simulink model "MobileManipulatorSlave"  (R2016a)
settings: Solver=FixedStepAuto  SolverMode=SingleTasking  StartTime=0.0  StopTime=inf  FixedStep=.001  RelTol=1e-3
undefined symbols (not defined in the file): DiscIntNeverNeededParam, transl
libraries: simulink x20, LibrarySimulinkSAS x2, dspfactors x1, aerolibanimutils x1, dspnetwork x1
(part 1 of 2)
settings Model: xpc_rtwmakecfg_data=_jpeg_  Creator=DSANTIAGO  LastModifiedBy=santd
settings DataIOCC: LimitDataPoints=on  SaveFormat=Array
settings OptimizationCC: BlockReduction=off  BooleanDataType=off
settings DebuggingCC: SaveWithParameterizedLinksMsg=none  UnderspecifiedInitializationDetection=Classic  MergeDetectMultiDrivingBlocksExec=none  SignalResolutionControl=TryResolveAllWithWarning  InvalidFcnCallConnMsg=warning  FcnCallInpInsideContextMsg=EnableAllAsWarning
settings HardwareCC: ProdBitPerPointer=32  ProdLargestAtomicFloat=None  ProdIntDivRoundTo=Undefined  ProdEndianess=Unspecified  ProdWordSize=32  ProdHWDeviceType=32-bit Generic  TargetUnknown=on
settings ModelReferenceCC: PropagateSignalLabelsOutOfModel=off
settings ConfigComp: CovSFcnEnable=off

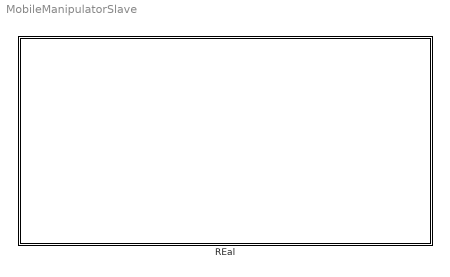
== system MobileManipulatorSlave ==
  "REal " : Subsystem  mask{sel=1, offSet=[1.5e-1 0 0.1]', h1=.01, h2=.01, kgmb=diag([8 10]), kgms=diag([4 4 4]), kms=10, kmb=5, ksb=1, ksm=diag([1 1 1])*2e3}
      mask prompts: sel "Control (s/m)"; h1 "Delay1"; h2 "Delay2"

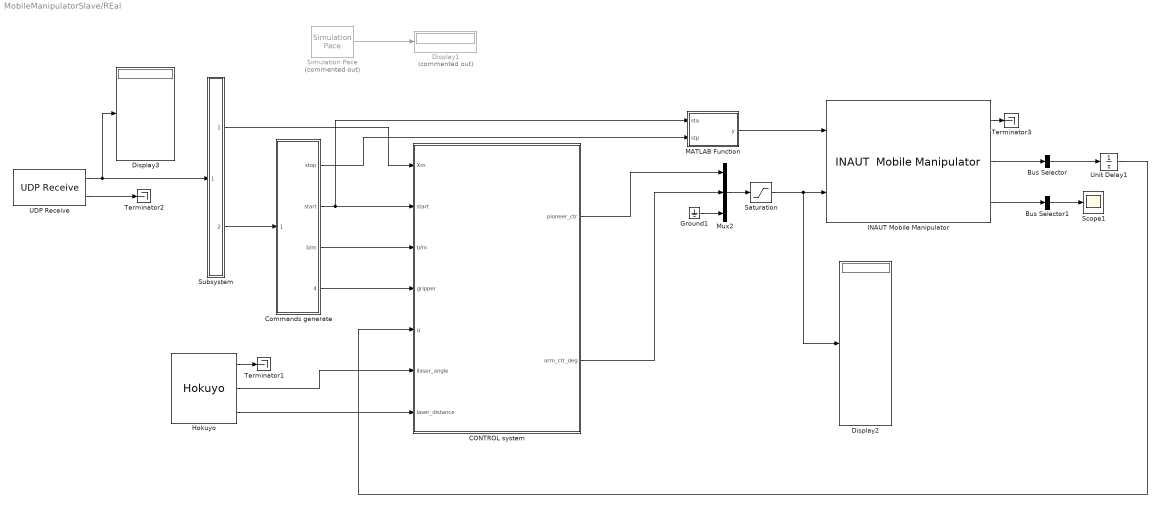
== system MobileManipulatorSlave/REal  ==
  Bus Selector : BusSelector  OutputSignals=q_{arm}  OutputAsBus=on
  Bus Selector1 : BusSelector  OutputSignals=base Info.current rigth motor?,base Info.current left motor?  OutputAsBus=on
  CONTROL system : Subsystem
  Commands generate : Subsystem
  Display1 : Display  Commented=on
  Display2 : Display
  Display3 : Display
  Ground1 : Ground
  Hokuyo : LibrarySimulinkSAS/Hokuyo
  INAUT Mobile Manipulator : LibrarySimulinkSAS/INAUT  Mobile Manipulator  IdB=3  IdM=1  IdL=0  ts=-1
  MATLAB Function : MATLAB Function  TreatAsAtomicUnit=on
  Mux2 : Mux  Inputs=3
  Saturation : Saturate  UpperLimit=2000  LowerLimit=-2000
  Scope1 : Scope
  Simulation Pace : aerolibanimutils/Simulation Pace  Commented=on  SimulationPace=1  SleepMode=MATLAB Thread  OutputPaceError=on  SampleTime=-1
  Subsystem : Subsystem
  Terminator1 : Terminator
  Terminator2 : Terminator
  Terminator3 : Terminator
  UDP Receive : dspnetwork/UDP Receive  localURL='0.0.0.0'  localPort=24100  remoteURL='0.0.0.0'  remotePort=-1  recvBufferSize=1024  dims=7  signalDatatype=double  isVarSize=off  showBlockingTime=off  blockingTime=0  sampletime=-1  blockPlatform=[]
  Unit Delay1 : UnitDelay  SampleTime=-1
  wires:
  Subsystem/1(xm) -> CONTROL system/1(Xm)
  Unit Delay1/1 -> CONTROL system/5(q)
  Subsystem/2(bt) -> Commands generate/1(butons)
  Commands generate/2(start) -> CONTROL system/2(start), MATLAB Function/1(sta)
  CONTROL system/2(arm_ctr_deg) -> Mux2/2
  Mux2/1 -> Saturation/1
  INAUT Mobile Manipulator/2 -> Bus Selector/1
  INAUT Mobile Manipulator/3 -> Bus Selector1/1
  INAUT Mobile Manipulator/1 -> Terminator3/1
  Bus Selector/1 -> Unit Delay1/1
  CONTROL system/1(pioneer_ctr) -> Mux2/1
  Ground1/1 -> Mux2/3
  Simulation Pace/1 -> Display1/1
  Commands generate/3(b/m) -> CONTROL system/3(b/m)
  Commands generate/4(griper) -> CONTROL system/4(gripper)
  UDP Receive/1 -> Subsystem/1(u), Display3/1
  UDP Receive/2 -> Terminator2/1
  Saturation/1 -> Display2/1, INAUT Mobile Manipulator/2
  Bus Selector1/1 -> Scope1/1
  MATLAB Function/1(y) -> INAUT Mobile Manipulator/1
  Commands generate/1(stop) -> MATLAB Function/2(stp)
  Hokuyo/1 -> Terminator1/1
  Hokuyo/2 -> CONTROL system/6(llaser_angle)
  Hokuyo/3 -> CONTROL system/7(laser_distance)

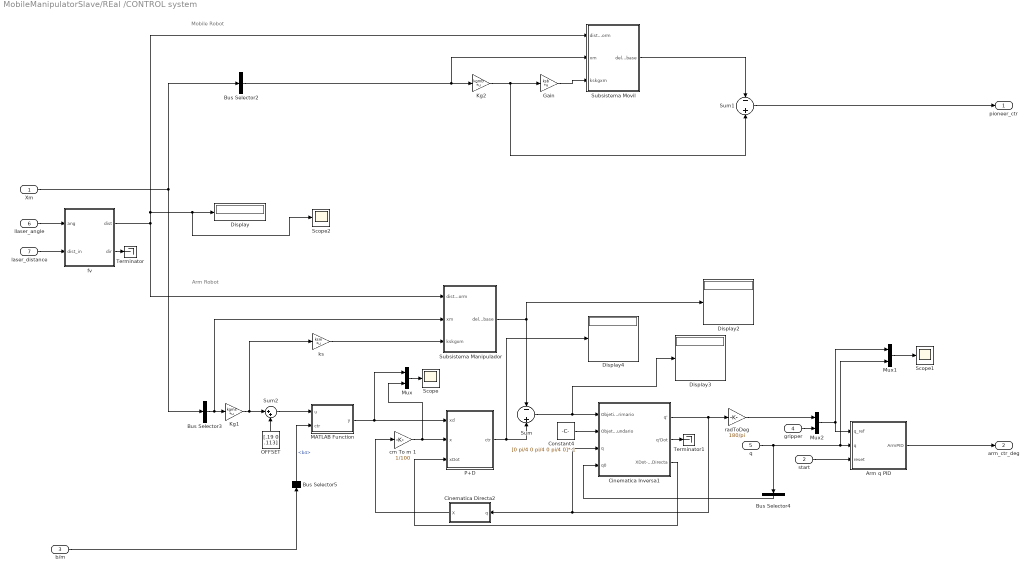
== system MobileManipulatorSlave/REal /CONTROL system ==
  note: Mobile Robot
  note: Arm Robot
  Xm : Inport
  start : Inport  Port=2
  b/m : Inport  Port=3
  gripper : Inport  Port=4
  q : Inport  Port=5
  llaser_angle : Inport  Port=6
  laser_distance : Inport  Port=7
  Arm q PID : Subsystem
  Bus Selector2 : BusSelector  OutputSignals=x,y  OutputAsBus=on
  Bus Selector3 : BusSelector  OutputSignals=x,y,z  OutputAsBus=on
  Bus Selector4 : BusSelector  OutputSignals=q1,q2,q3,q4,q5,q6,q7  OutputAsBus=on
  Bus Selector5 : BusSelector  OutputSignals=b4
  Cinematica Directa2 : Subsystem
  Cinematica Inversa1 : Subsystem
  Constant4 : Constant  Value=[0 pi/4 0 pi/4 0 pi/4 0]*-1
  Display{,2..4} (4 alike) : Display
  Gain : Gain  Gain=ksb  Multiplication=Matrix(K*u)
  Kg1 : Gain  Gain=kgms  Multiplication=Matrix(K*u)
  Kg2 : Gain  Gain=kgmb  Multiplication=Matrix(K*u)
  MATLAB Function : MATLAB Function  TreatAsAtomicUnit=on
  Mux : Mux  Inputs=2
  Mux1 : Mux  Inputs=2
  Mux2 : Mux  Inputs=2
  OFFSET : Constant  Value=[.19 0 .113]
  P+D : Subsystem
  Scope : Scope
  Scope1 : Scope
  Scope2 : Scope
  Subsistema Manipulador : Subsystem
  Subsistema Movil : Subsystem
  Sum : Sum  Inputs=-+
  Sum1 : Sum  Inputs=-+
  Sum2 : Sum  Inputs=|++
  Terminator : Terminator
  Terminator1 : Terminator
  cm To m 1 : Gain  Gain=1/100
  fv : Subsystem
  ks : Gain  Gain=ksm  Multiplication=Matrix(K*u)
  radToDeg : Gain  Gain=180/pi
  pioneer_ctr : Outport
  arm_ctr_deg : Outport  Port=2
  wires:
  Xm/1 -> Bus Selector3/1, Bus Selector2/1
  Bus Selector2/1 -> Subsistema Movil/2(xm), Kg2/1
  Cinematica Inversa1/1(q') -> Cinematica Inversa1/3(q), Cinematica Directa2/1(q), radToDeg/1
  OFFSET/1 -> Sum2/2
  Kg1/1 -> ks/1, Sum2/1
  P+D/1(ctr) -> Display4/1, Sum/2
  Cinematica Directa2/1("X ") -> cm To m 1/1
  cm To m 1/1 -> Mux/2, P+D/2(x)
  Constant4/1 -> Cinematica Inversa1/2(Objetivo Secundario)
  gripper/1 -> Mux2/2
  start/1 -> Arm q PID/3(reset)
  b/m/1 -> Bus Selector5/1
  Kg2/1 -> Sum1/2, Gain/1
  radToDeg/1 -> Mux2/1
  Sum2/1 -> MATLAB Function/1(u)
  Cinematica Inversa1/2(q'Dot) -> Terminator1/1
  Mux/1 -> Scope/1
  Cinematica Inversa1/3(XDot- CinematicaDirecta) -> P+D/3(xDot)
  q/1 -> Bus Selector4/1, Mux1/2, Arm q PID/2(q)
  Mux2/1 -> Mux1/1, Arm q PID/1(q_ref)
  Mux1/1 -> Scope1/1
  Bus Selector4/1 -> Cinematica Inversa1/4(q0)
  MATLAB Function/1(y) -> P+D/1(xd), Mux/1
  Bus Selector5/1 -> MATLAB Function/2(ctr)  "<b4>"
  Arm q PID/1(ArmPID) -> arm_ctr_deg/1
  Gain/1 -> Subsistema Movil/3(kskgxm)
  Subsistema Movil/1(delta_base) -> Sum1/1
  fv/2(dir) -> Terminator/1
  laser_distance/1 -> fv/2(dist_in)
  llaser_angle/1 -> fv/1(ang)
  fv/1(dist) -> Subsistema Manipulador/1(dist_norm), Scope2/1, Display/1, Subsistema Movil/1(dist_norm)
  Subsistema Manipulador/1(delta_base) -> Display2/1, Sum/1
  Sum/1 -> Display3/1, Cinematica Inversa1/1(Objetivo Primario)
  Bus Selector3/1 -> Subsistema Manipulador/2(xm), Kg1/1
  ks/1 -> Subsistema Manipulador/3(kskgxm)
  Sum1/1 -> pioneer_ctr/1

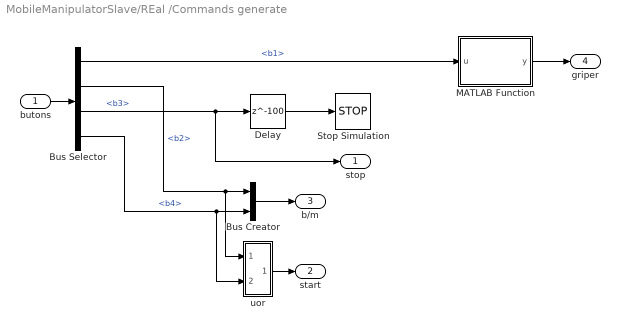
== system MobileManipulatorSlave/REal /Commands generate ==
  butons : Inport
  Bus Creator : BusCreator  Inputs=2
  Bus Selector : BusSelector  OutputSignals=b1,b2,b3,b4
  Delay : Delay  DelayLength=100
  MATLAB Function : MATLAB Function  TreatAsAtomicUnit=on
  Stop Simulation : Stop
  uor : Subsystem
  stop : Outport
  start : Outport  Port=2
  b/m : Outport  Port=3
  griper : Outport  Port=4
  wires:
  Bus Selector/2 -> uor/1(u1), Bus Creator/1  "<b2>"
  Bus Selector/3 -> stop/1, Delay/1  "<b3>"
  Delay/1 -> Stop Simulation/1
  Bus Creator/1 -> b/m/1
  Bus Selector/4 -> uor/2(u2), Bus Creator/2  "<b4>"
  Bus Selector/1 -> MATLAB Function/1(u)  "<b1>"
  butons/1 -> Bus Selector/1
  uor/1(y) -> start/1
  MATLAB Function/1(y) -> griper/1

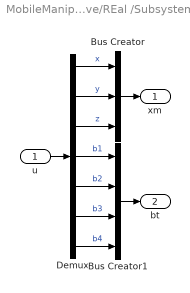
== system MobileManipulatorSlave/REal /Subsystem ==
  u : Inport
  Bus Creator : BusCreator  Inputs=3
  Bus Creator1 : BusCreator  Inputs=4
  Demux : Demux  Outputs=7
  xm : Outport
  bt : Outport  Port=2
  wires:
  Demux/2 -> Bus Creator/2  "y"
  Demux/3 -> Bus Creator/3  "z"
  Demux/5 -> Bus Creator1/2  "b2"
  Demux/1 -> Bus Creator/1  "x"
  Demux/6 -> Bus Creator1/3  "b3"
  Demux/4 -> Bus Creator1/1  "b1"
  Demux/7 -> Bus Creator1/4  "b4"
  Bus Creator1/1 -> bt/1
  u/1 -> Demux/1
  Bus Creator/1 -> xm/1

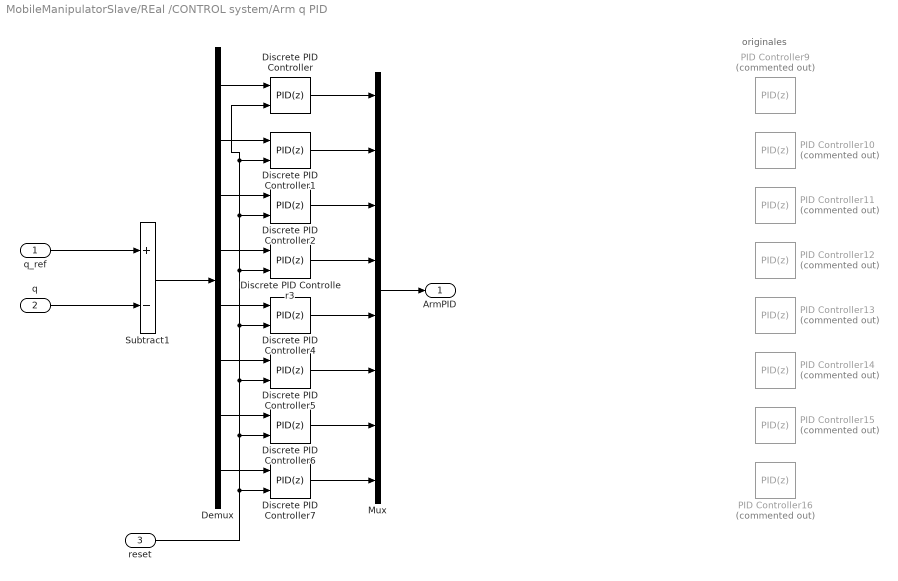
== system MobileManipulatorSlave/REal /CONTROL system/Arm q PID ==
  note: originales
  q_ref : Inport
  q : Inport  Port=2
  reset : Inport  Port=3
  Demux : Demux  Outputs=8
  Discrete PID Controlle r3 : simulink/Continuous/PID Controller  Controller=PID  TimeDomain=Discrete-time  SampleTime=-1  IntegratorMethod=Forward Euler  FilterMethod=Forward Euler  Form=Parallel  UseFilter=on  ControllerParametersSource=internal  P=75  I=40  D=0.01  N=100  InitialConditionSource=internal  InitialConditionForIntegrator=0  InitialConditionForFilter=0  ExternalReset=level  LimitOutput=on  UpperSaturationLimit=4095  LowerSaturationLimit=-4095  LinearizeAsGain=on  AntiWindupMode=clamping  Kb=1  TrackingMode=off  Kt=1  PParamMin=[]  PParamMax=[]  IParamMin=[]  IParamMax=[]  DParamMin=[]  DParamMax=[]  NParamMin=[]  NParamMax=[]  KbParamMin=[]  KbParamMax=[]  KtParamMin=[]  KtParamMax=[]  POutMin=[]  POutMax=[]  IOutMin=[]  IOutMax=[]  DOutMin=[]  DOutMax=[]  NOutMin=[]  NOutMax=[]  KbOutMin=[]  KbOutMax=[]  KtOutMin=[]  KtOutMax=[]  IntegratorOutMin=[]  IntegratorOutMax=[]  FilterOutMin=[]  FilterOutMax=[]  SumOutMin=[]  SumOutMax=[]  SumI1OutMin=[]  SumI1OutMax=[]  SumI2OutMin=[]  SumI2OutMax=[]  SumI3OutMin=[]  SumI3OutMax=[]  SumDOutMin=[]  SumDOutMax=[]  SaturationOutMin=[]  SaturationOutMax=[]  IntegratorContinuousStateAttributes=''  IntegratorStateMustResolveToSignalObject=off  IntegratorRTWStateStorageClass=Auto  FilterContinuousStateAttributes=''  FilterStateMustResolveToSignalObject=off  FilterRTWStateStorageClass=Auto  DifferentiatorICPrevScaledInput=0  DifferentiatorOutMin=[]  DifferentiatorOutMax=[]
  Discrete PID Controller : simulink/Continuous/PID Controller  Controller=PID  TimeDomain=Discrete-time  SampleTime=-1  IntegratorMethod=Forward Euler  FilterMethod=Forward Euler  Form=Parallel  UseFilter=on  ControllerParametersSource=internal  P=125  I=40  D=0.01  N=100  InitialConditionSource=internal  InitialConditionForIntegrator=0  InitialConditionForFilter=0  ExternalReset=level  LimitOutput=on  UpperSaturationLimit=4095  LowerSaturationLimit=-4095  LinearizeAsGain=on  AntiWindupMode=clamping  Kb=1  TrackingMode=off  Kt=1  PParamMin=[]  PParamMax=[]  IParamMin=[]  IParamMax=[]  DParamMin=[]  DParamMax=[]  NParamMin=[]  NParamMax=[]  KbParamMin=[]  KbParamMax=[]  KtParamMin=[]  KtParamMax=[]  POutMin=[]  POutMax=[]  IOutMin=[]  IOutMax=[]  DOutMin=[]  DOutMax=[]  NOutMin=[]  NOutMax=[]  KbOutMin=[]  KbOutMax=[]  KtOutMin=[]  KtOutMax=[]  IntegratorOutMin=[]  IntegratorOutMax=[]  FilterOutMin=[]  FilterOutMax=[]  SumOutMin=[]  SumOutMax=[]  SumI1OutMin=[]  SumI1OutMax=[]  SumI2OutMin=[]  SumI2OutMax=[]  SumI3OutMin=[]  SumI3OutMax=[]  SumDOutMin=[]  SumDOutMax=[]  SaturationOutMin=[]  SaturationOutMax=[]  IntegratorContinuousStateAttributes=''  IntegratorStateMustResolveToSignalObject=off  IntegratorRTWStateStorageClass=Auto  FilterContinuousStateAttributes=''  FilterStateMustResolveToSignalObject=off  FilterRTWStateStorageClass=Auto  DifferentiatorICPrevScaledInput=0  DifferentiatorOutMin=[]  DifferentiatorOutMax=[]
  Discrete PID Controller1 : simulink/Continuous/PID Controller  Controller=PID  TimeDomain=Discrete-time  SampleTime=-1  IntegratorMethod=Forward Euler  FilterMethod=Forward Euler  Form=Parallel  UseFilter=on  ControllerParametersSource=internal  P=75  I=100  D=0.01  N=100  InitialConditionSource=internal  InitialConditionForIntegrator=0  InitialConditionForFilter=0  ExternalReset=level  LimitOutput=on  UpperSaturationLimit=4095  LowerSaturationLimit=-4095  LinearizeAsGain=on  AntiWindupMode=clamping  Kb=1  TrackingMode=off  Kt=1  PParamMin=[]  PParamMax=[]  IParamMin=[]  IParamMax=[]  DParamMin=[]  DParamMax=[]  NParamMin=[]  NParamMax=[]  KbParamMin=[]  KbParamMax=[]  KtParamMin=[]  KtParamMax=[]  POutMin=[]  POutMax=[]  IOutMin=[]  IOutMax=[]  DOutMin=[]  DOutMax=[]  NOutMin=[]  NOutMax=[]  KbOutMin=[]  KbOutMax=[]  KtOutMin=[]  KtOutMax=[]  IntegratorOutMin=[]  IntegratorOutMax=[]  FilterOutMin=[]  FilterOutMax=[]  SumOutMin=[]  SumOutMax=[]  SumI1OutMin=[]  SumI1OutMax=[]  SumI2OutMin=[]  SumI2OutMax=[]  SumI3OutMin=[]  SumI3OutMax=[]  SumDOutMin=[]  SumDOutMax=[]  SaturationOutMin=[]  SaturationOutMax=[]  IntegratorContinuousStateAttributes=''  IntegratorStateMustResolveToSignalObject=off  IntegratorRTWStateStorageClass=Auto  FilterContinuousStateAttributes=''  FilterStateMustResolveToSignalObject=off  FilterRTWStateStorageClass=Auto  DifferentiatorICPrevScaledInput=0  DifferentiatorOutMin=[]  DifferentiatorOutMax=[]
  Discrete PID Controller2 : simulink/Continuous/PID Controller  Controller=PID  TimeDomain=Discrete-time  SampleTime=-1  IntegratorMethod=Forward Euler  FilterMethod=Forward Euler  Form=Parallel  UseFilter=on  ControllerParametersSource=internal  P=80  I=45  D=0.01  N=100  InitialConditionSource=internal  InitialConditionForIntegrator=0  InitialConditionForFilter=0  ExternalReset=level  LimitOutput=on  UpperSaturationLimit=4095  LowerSaturationLimit=-4095  LinearizeAsGain=on  AntiWindupMode=clamping  Kb=1  TrackingMode=off  Kt=1  PParamMin=[]  PParamMax=[]  IParamMin=[]  IParamMax=[]  DParamMin=[]  DParamMax=[]  NParamMin=[]  NParamMax=[]  KbParamMin=[]  KbParamMax=[]  KtParamMin=[]  KtParamMax=[]  POutMin=[]  POutMax=[]  IOutMin=[]  IOutMax=[]  DOutMin=[]  DOutMax=[]  NOutMin=[]  NOutMax=[]  KbOutMin=[]  KbOutMax=[]  KtOutMin=[]  KtOutMax=[]  IntegratorOutMin=[]  IntegratorOutMax=[]  FilterOutMin=[]  FilterOutMax=[]  SumOutMin=[]  SumOutMax=[]  SumI1OutMin=[]  SumI1OutMax=[]  SumI2OutMin=[]  SumI2OutMax=[]  SumI3OutMin=[]  SumI3OutMax=[]  SumDOutMin=[]  SumDOutMax=[]  SaturationOutMin=[]  SaturationOutMax=[]  IntegratorContinuousStateAttributes=''  IntegratorStateMustResolveToSignalObject=off  IntegratorRTWStateStorageClass=Auto  FilterContinuousStateAttributes=''  FilterStateMustResolveToSignalObject=off  FilterRTWStateStorageClass=Auto  DifferentiatorICPrevScaledInput=0  DifferentiatorOutMin=[]  DifferentiatorOutMax=[]
  Discrete PID Controller{4..7} (4 alike) : simulink/Continuous/PID Controller  Controller=PID  TimeDomain=Discrete-time  SampleTime=-1  IntegratorMethod=Forward Euler  FilterMethod=Forward Euler  Form=Parallel  UseFilter=on  ControllerParametersSource=internal  P=75  I=40  D=0.01  N=100  InitialConditionSource=internal  InitialConditionForIntegrator=0  InitialConditionForFilter=0  ExternalReset=level  LimitOutput=on  UpperSaturationLimit=4095  LowerSaturationLimit=-4095  LinearizeAsGain=on  AntiWindupMode=clamping  Kb=1  TrackingMode=off  Kt=1  PParamMin=[]  PParamMax=[]  IParamMin=[]  IParamMax=[]  DParamMin=[]  DParamMax=[]  NParamMin=[]  NParamMax=[]  KbParamMin=[]  KbParamMax=[]  KtParamMin=[]  KtParamMax=[]  POutMin=[]  POutMax=[]  IOutMin=[]  IOutMax=[]  DOutMin=[]  DOutMax=[]  NOutMin=[]  NOutMax=[]  KbOutMin=[]  KbOutMax=[]  KtOutMin=[]  KtOutMax=[]  IntegratorOutMin=[]  IntegratorOutMax=[]  FilterOutMin=[]  FilterOutMax=[]  SumOutMin=[]  SumOutMax=[]  SumI1OutMin=[]  SumI1OutMax=[]  SumI2OutMin=[]  SumI2OutMax=[]  SumI3OutMin=[]  SumI3OutMax=[]  SumDOutMin=[]  SumDOutMax=[]  SaturationOutMin=[]  SaturationOutMax=[]  IntegratorContinuousStateAttributes=''  IntegratorStateMustResolveToSignalObject=off  IntegratorRTWStateStorageClass=Auto  FilterContinuousStateAttributes=''  FilterStateMustResolveToSignalObject=off  FilterRTWStateStorageClass=Auto  DifferentiatorICPrevScaledInput=0  DifferentiatorOutMin=[]  DifferentiatorOutMax=[]
  Mux : Mux  Inputs=8
  PID Controller10 : simulink/Continuous/PID Controller  Commented=on  Controller=PID  TimeDomain=Discrete-time  SampleTime=-1  IntegratorMethod=Forward Euler  FilterMethod=Forward Euler  Form=Parallel  UseFilter=on  ControllerParametersSource=internal  P=75  I=100  D=0.01  N=100  InitialConditionSource=internal  InitialConditionForIntegrator=0  InitialConditionForFilter=0  ExternalReset=rising  LimitOutput=on  UpperSaturationLimit=4095  LowerSaturationLimit=-4095  LinearizeAsGain=on  AntiWindupMode=clamping  Kb=1  TrackingMode=off  Kt=1  PParamMin=[]  PParamMax=[]  PParamDataTypeStr=single  IParamMin=[]  IParamMax=[]  IParamDataTypeStr=single  DParamMin=[]  DParamMax=[]  DParamDataTypeStr=single  NParamMin=[]  NParamMax=[]  NParamDataTypeStr=single  KbParamMin=[]  KbParamMax=[]  KtParamMin=[]  KtParamMax=[]  POutMin=[]  POutMax=[]  POutDataTypeStr=single  PGainOutDataTypeStr=single  PProdOutDataTypeStr=single  IOutMin=[]  IOutMax=[]  IOutDataTypeStr=single  IGainOutDataTypeStr=single  IProdOutDataTypeStr=single  DOutMin=[]  DOutMax=[]  DOutDataTypeStr=single  DGainOutDataTypeStr=single  DProdOutDataTypeStr=single  NOutMin=[]  NOutMax=[]  NOutDataTypeStr=single  NGainOutDataTypeStr=single  NProdOutDataTypeStr=single  KbOutMin=[]  KbOutMax=[]  KtOutMin=[]  KtOutMax=[]  IntegratorOutMin=[]  IntegratorOutMax=[]  IntegratorOutDataTypeStr=single  FilterOutMin=[]  FilterOutMax=[]  FilterOutDataTypeStr=single  SumOutMin=[]  SumOutMax=[]  SumOutDataTypeStr=single  SumI1OutMin=[]  SumI1OutMax=[]  SumI2OutMin=[]  SumI2OutMax=[]  SumI3OutMin=[]  SumI3OutMax=[]  SumDOutMin=[]  SumDOutMax=[]  SumDOutDataTypeStr=single  SumAccumDataTypeStr=single  SumDAccumDataTypeStr=single  SaturationOutMin=[]  SaturationOutMax=[]  SaturationOutDataTypeStr=single  IntegratorContinuousStateAttributes=''  IntegratorStateMustResolveToSignalObject=off  IntegratorRTWStateStorageClass=Auto  FilterContinuousStateAttributes=''  FilterStateMustResolveToSignalObject=off  FilterRTWStateStorageClass=Auto  DifferentiatorICPrevScaledInput=0  DifferentiatorOutMin=[]  DifferentiatorOutMax=[]
  PID Controller11 : simulink/Continuous/PID Controller  Commented=on  Controller=PID  TimeDomain=Discrete-time  SampleTime=-1  IntegratorMethod=Forward Euler  FilterMethod=Forward Euler  Form=Parallel  UseFilter=on  ControllerParametersSource=internal  P=80  I=45  D=0.01  N=100  InitialConditionSource=internal  InitialConditionForIntegrator=0  InitialConditionForFilter=0  ExternalReset=rising  LimitOutput=on  UpperSaturationLimit=4095  LowerSaturationLimit=-4095  LinearizeAsGain=on  AntiWindupMode=clamping  Kb=1  TrackingMode=off  Kt=1  PParamMin=[]  PParamMax=[]  PParamDataTypeStr=single  IParamMin=[]  IParamMax=[]  IParamDataTypeStr=single  DParamMin=[]  DParamMax=[]  DParamDataTypeStr=single  NParamMin=[]  NParamMax=[]  NParamDataTypeStr=single  KbParamMin=[]  KbParamMax=[]  KtParamMin=[]  KtParamMax=[]  POutMin=[]  POutMax=[]  POutDataTypeStr=single  PGainOutDataTypeStr=single  PProdOutDataTypeStr=single  IOutMin=[]  IOutMax=[]  IOutDataTypeStr=single  IGainOutDataTypeStr=single  IProdOutDataTypeStr=single  DOutMin=[]  DOutMax=[]  DOutDataTypeStr=single  DGainOutDataTypeStr=single  DProdOutDataTypeStr=single  NOutMin=[]  NOutMax=[]  NOutDataTypeStr=single  NGainOutDataTypeStr=single  NProdOutDataTypeStr=single  KbOutMin=[]  KbOutMax=[]  KtOutMin=[]  KtOutMax=[]  IntegratorOutMin=[]  IntegratorOutMax=[]  IntegratorOutDataTypeStr=single  FilterOutMin=[]  FilterOutMax=[]  FilterOutDataTypeStr=single  SumOutMin=[]  SumOutMax=[]  SumOutDataTypeStr=single  SumI1OutMin=[]  SumI1OutMax=[]  SumI2OutMin=[]  SumI2OutMax=[]  SumI3OutMin=[]  SumI3OutMax=[]  SumDOutMin=[]  SumDOutMax=[]  SumDOutDataTypeStr=single  SumAccumDataTypeStr=single  SumDAccumDataTypeStr=single  SaturationOutMin=[]  SaturationOutMax=[]  SaturationOutDataTypeStr=single  IntegratorContinuousStateAttributes=''  IntegratorStateMustResolveToSignalObject=off  IntegratorRTWStateStorageClass=Auto  FilterContinuousStateAttributes=''  FilterStateMustResolveToSignalObject=off  FilterRTWStateStorageClass=Auto  DifferentiatorICPrevScaledInput=0  DifferentiatorOutMin=[]  DifferentiatorOutMax=[]
  PID Controller{12..16} (5 alike) : simulink/Continuous/PID Controller  Commented=on  Controller=PID  TimeDomain=Discrete-time  SampleTime=-1  IntegratorMethod=Forward Euler  FilterMethod=Forward Euler  Form=Parallel  UseFilter=on  ControllerParametersSource=internal  P=75  I=40  D=0.01  N=100  InitialConditionSource=internal  InitialConditionForIntegrator=0  InitialConditionForFilter=0  ExternalReset=rising  LimitOutput=on  UpperSaturationLimit=4095  LowerSaturationLimit=-4095  LinearizeAsGain=on  AntiWindupMode=clamping  Kb=1  TrackingMode=off  Kt=1  PParamMin=[]  PParamMax=[]  PParamDataTypeStr=single  IParamMin=[]  IParamMax=[]  IParamDataTypeStr=single  DParamMin=[]  DParamMax=[]  DParamDataTypeStr=single  NParamMin=[]  NParamMax=[]  NParamDataTypeStr=single  KbParamMin=[]  KbParamMax=[]  KtParamMin=[]  KtParamMax=[]  POutMin=[]  POutMax=[]  POutDataTypeStr=single  PGainOutDataTypeStr=single  PProdOutDataTypeStr=single  IOutMin=[]  IOutMax=[]  IOutDataTypeStr=single  IGainOutDataTypeStr=single  IProdOutDataTypeStr=single  DOutMin=[]  DOutMax=[]  DOutDataTypeStr=single  DGainOutDataTypeStr=single  DProdOutDataTypeStr=single  NOutMin=[]  NOutMax=[]  NOutDataTypeStr=single  NGainOutDataTypeStr=single  NProdOutDataTypeStr=single  KbOutMin=[]  KbOutMax=[]  KtOutMin=[]  KtOutMax=[]  IntegratorOutMin=[]  IntegratorOutMax=[]  IntegratorOutDataTypeStr=single  FilterOutMin=[]  FilterOutMax=[]  FilterOutDataTypeStr=single  SumOutMin=[]  SumOutMax=[]  SumOutDataTypeStr=single  SumI1OutMin=[]  SumI1OutMax=[]  SumI2OutMin=[]  SumI2OutMax=[]  SumI3OutMin=[]  SumI3OutMax=[]  SumDOutMin=[]  SumDOutMax=[]  SumDOutDataTypeStr=single  SumAccumDataTypeStr=single  SumDAccumDataTypeStr=single  SaturationOutMin=[]  SaturationOutMax=[]  SaturationOutDataTypeStr=single  IntegratorContinuousStateAttributes=''  IntegratorStateMustResolveToSignalObject=off  IntegratorRTWStateStorageClass=Auto  FilterContinuousStateAttributes=''  FilterStateMustResolveToSignalObject=off  FilterRTWStateStorageClass=Auto  DifferentiatorICPrevScaledInput=0  DifferentiatorOutMin=[]  DifferentiatorOutMax=[]
  PID Controller9 : simulink/Continuous/PID Controller  Commented=on  Controller=PID  TimeDomain=Discrete-time  SampleTime=-1  IntegratorMethod=Forward Euler  FilterMethod=Forward Euler  Form=Parallel  UseFilter=on  ControllerParametersSource=internal  P=125  I=40  D=0.01  N=100  InitialConditionSource=internal  InitialConditionForIntegrator=0  InitialConditionForFilter=0  ExternalReset=level  LimitOutput=on  UpperSaturationLimit=4095  LowerSaturationLimit=-4095  LinearizeAsGain=on  AntiWindupMode=clamping  Kb=1  TrackingMode=off  Kt=1  PParamMin=[]  PParamMax=[]  PParamDataTypeStr=single  IParamMin=[]  IParamMax=[]  IParamDataTypeStr=single  DParamMin=[]  DParamMax=[]  DParamDataTypeStr=single  NParamMin=[]  NParamMax=[]  NParamDataTypeStr=single  KbParamMin=[]  KbParamMax=[]  KtParamMin=[]  KtParamMax=[]  POutMin=[]  POutMax=[]  POutDataTypeStr=single  PGainOutDataTypeStr=single  PProdOutDataTypeStr=single  IOutMin=[]  IOutMax=[]  IOutDataTypeStr=single  IGainOutDataTypeStr=single  IProdOutDataTypeStr=single  DOutMin=[]  DOutMax=[]  DOutDataTypeStr=single  DGainOutDataTypeStr=single  DProdOutDataTypeStr=single  NOutMin=[]  NOutMax=[]  NOutDataTypeStr=single  NGainOutDataTypeStr=single  NProdOutDataTypeStr=single  KbOutMin=[]  KbOutMax=[]  KtOutMin=[]  KtOutMax=[]  IntegratorOutMin=[]  IntegratorOutMax=[]  IntegratorOutDataTypeStr=single  FilterOutMin=[]  FilterOutMax=[]  FilterOutDataTypeStr=single  SumOutMin=[]  SumOutMax=[]  SumOutDataTypeStr=single  SumI1OutMin=[]  SumI1OutMax=[]  SumI2OutMin=[]  SumI2OutMax=[]  SumI3OutMin=[]  SumI3OutMax=[]  SumDOutMin=[]  SumDOutMax=[]  SumDOutDataTypeStr=single  SumAccumDataTypeStr=single  SumDAccumDataTypeStr=single  SaturationOutMin=[]  SaturationOutMax=[]  SaturationOutDataTypeStr=single  IntegratorContinuousStateAttributes=''  IntegratorStateMustResolveToSignalObject=off  IntegratorRTWStateStorageClass=Auto  FilterContinuousStateAttributes=''  FilterStateMustResolveToSignalObject=off  FilterRTWStateStorageClass=Auto  DifferentiatorICPrevScaledInput=0  DifferentiatorOutMin=[]  DifferentiatorOutMax=[]
  Subtract1 : Sum  Inputs=+-
  ArmPID : Outport  PortDimensions=8
  wires:
  q/1 -> Subtract1/2
  q_ref/1 -> Subtract1/1
  Demux/1 -> Discrete PID Controller/1
  Subtract1/1 -> Demux/1
  Demux/6 -> Discrete PID Controller5/1
  Demux/2 -> Discrete PID Controller1/1
  Demux/3 -> Discrete PID Controller2/1
  Demux/4 -> Discrete PID Controlle r3/1
  Demux/5 -> Discrete PID Controller4/1
  Demux/7 -> Discrete PID Controller6/1
  Demux/8 -> Discrete PID Controller7/1
  Discrete PID Controller7/1 -> Mux/8
  Discrete PID Controller6/1 -> Mux/7
  Discrete PID Controller5/1 -> Mux/6
  Discrete PID Controller4/1 -> Mux/5
  Discrete PID Controlle r3/1 -> Mux/4
  Discrete PID Controller2/1 -> Mux/3
  Discrete PID Controller1/1 -> Mux/2
  reset/1 -> Discrete PID Controller7/2, Discrete PID Controller6/2, Discrete PID Controller5/2, Discrete PID Controller4/2, Discrete PID Controlle r3/2, Discrete PID Controller2/2, Discrete PID Controller1/2, Discrete PID Controller/2
  Discrete PID Controller/1 -> Mux/1
  Mux/1 -> ArmPID/1

== system MobileManipulatorSlave/REal /CONTROL system/Cinematica Directa2 ==
  q : Inport
  Mux1 : Mux  Inputs=3
  T2xyz1 : Subsystem
      mask help: Convert transform to xyz scalars
      mask Help:
      | Convert homogeneous transformation to position scalars.
      | 
      | 
      | <b>Inputs::</b>
      | 
      | T (4x4) a translation represented as a homogeneous transformation
      | 
      | <b>Outputs::</b>
      | 
      | x (1x1) x-coordinate
      | y (1x1) y-coordinate
      | z (1x1) z-coordinate
      | 
      | <b>Notes::</b>
      | 
      | - A wrapper for the Toolbox function transl().
  fkine in [cm] : MATLAB Function  TreatAsAtomicUnit=on
  "X " : Outport
  wires:
  fkine in [cm]/1(out1) -> T2xyz1/1(T)
  Mux1/1 -> "X "/1
  T2xyz1/1(x) -> Mux1/1
  T2xyz1/2(y) -> Mux1/2
  T2xyz1/3(z) -> Mux1/3
  q/1 -> fkine in [cm]/1(in1)

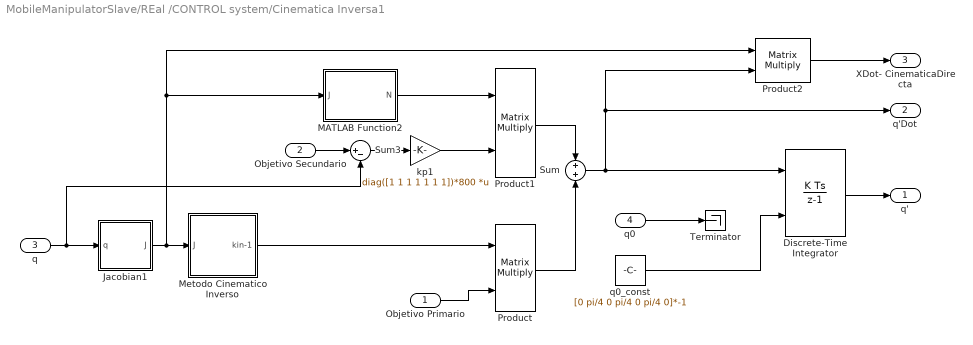
== system MobileManipulatorSlave/REal /CONTROL system/Cinematica Inversa1 ==
  Objetivo Primario : Inport
  Objetivo Secundario : Inport  Port=2
  q : Inport  Port=3
  q0 : Inport  Port=4
  Discrete-Time Integrator : DiscreteIntegrator  InitialConditionSource=external  InitialConditionSetting=State (most efficient)  SampleTime=-1  ICPrevOutput=DiscIntNeverNeededParam  ICPrevScaledInput=DiscIntNeverNeededParam
  Jacobian1 : Subsystem
  MATLAB Function2 : MATLAB Function  TreatAsAtomicUnit=on
  Metodo Cinematico Inverso : Subsystem
  Product : Product  Multiplication=Matrix(*)
  Product1 : Product  Multiplication=Matrix(*)
  Product2 : Product  Multiplication=Matrix(*)
  Sum : Sum
  Sum3 : Sum  Inputs=|+-
  Terminator : Terminator
  kp1 : Gain  Gain=diag([1 1 1 1 1 1 1])*800  Multiplication=Matrix(K*u)
  q0_const : Constant  Value=[0 pi/4 0 pi/4 0 pi/4 0]*-1
  q' : Outport
  q'Dot : Outport  Port=2
  XDot- CinematicaDirecta : Outport  Port=3
  wires:
  MATLAB Function2/1(N) -> Product1/1
  Product1/1 -> Sum/1
  Sum/1 -> Discrete-Time Integrator/1, Product2/2, q'Dot/1
  Product/1 -> Sum/2
  q/1 -> Sum3/2, Jacobian1/1(q)
  Jacobian1/1(J) -> MATLAB Function2/1(J), Product2/1, Metodo Cinematico Inverso/1(J)
  Objetivo Secundario/1 -> Sum3/1
  Sum3/1 -> kp1/1
  kp1/1 -> Product1/2
  Discrete-Time Integrator/1 -> q'/1
  Metodo Cinematico Inverso/1(kin-1) -> Product/1
  Objetivo Primario/1 -> Product/2
  Product2/1 -> XDot- CinematicaDirecta/1
  q0/1 -> Terminator/1
  q0_const/1 -> Discrete-Time Integrator/2

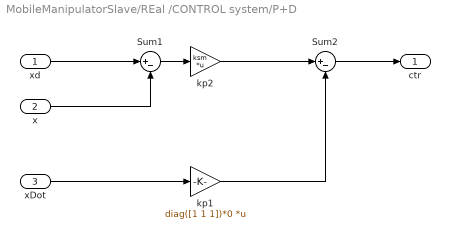
== system MobileManipulatorSlave/REal /CONTROL system/P+D ==
  xd : Inport
  x : Inport  Port=2
  xDot : Inport  Port=3
  Sum1 : Sum  Inputs=|+-
  Sum2 : Sum  Inputs=|+-
  kp1 : Gain  Gain=diag([1 1 1])*0  Multiplication=Matrix(K*u)
  kp2 : Gain  Gain=ksm  Multiplication=Matrix(K*u)
  ctr : Outport
  wires:
  x/1 -> Sum1/2
  xd/1 -> Sum1/1
  Sum2/1 -> ctr/1
  Sum1/1 -> kp2/1
  xDot/1 -> kp1/1
  kp2/1 -> Sum2/1
  kp1/1 -> Sum2/2

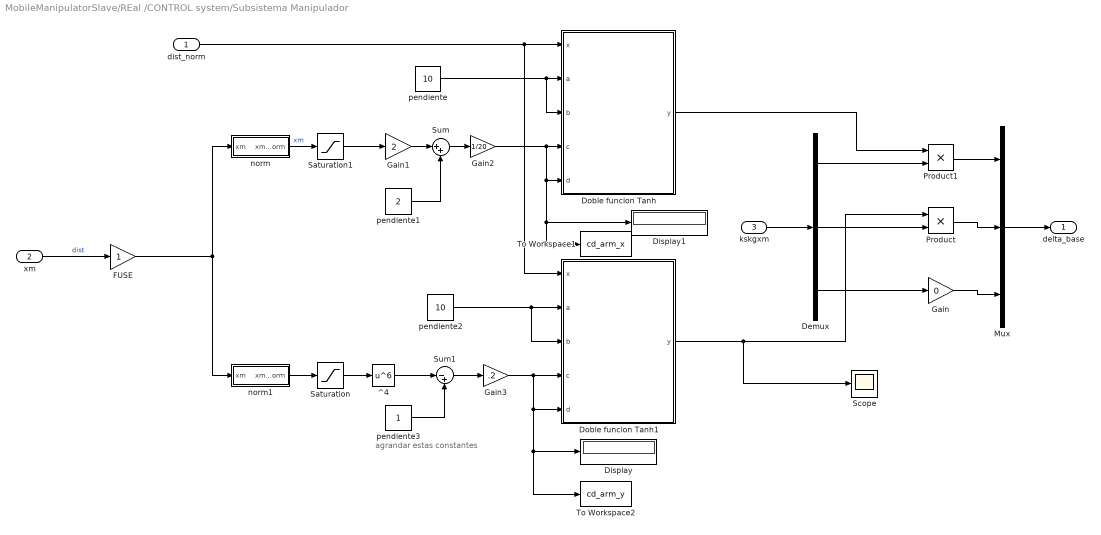
== system MobileManipulatorSlave/REal /CONTROL system/Subsistema Manipulador ==
  note: agrandar estas constantes
  dist_norm : Inport
  xm : Inport  Port=2
  kskgxm : Inport  Port=3
  Demux : Demux  Outputs=3
  Display : Display
  Display1 : Display
  Doble funcion Tanh : MATLAB Function  TreatAsAtomicUnit=on
  Doble funcion Tanh1 : MATLAB Function  TreatAsAtomicUnit=on
  FUSE : Gain
  Gain : Gain  Gain=0
  Gain1 : Gain  Gain=2
  Gain2 : Gain  Gain=1/20
  Gain3 : Gain  Gain=.2
  Mux : Mux  Inputs=3
  Product : Product
  Product1 : Product
  Saturation : Saturate  UpperLimit=1  LowerLimit=-1
  Saturation1 : Saturate  UpperLimit=1  LowerLimit=-1
  Scope : Scope
  Sum : Sum  Inputs=|++
  Sum1 : Sum  Inputs=|-+
  To Workspace1 : ToWorkspace  VariableName=cd_arm_x  SaveFormat=Timeseries  SampleTime=-1
  To Workspace2 : ToWorkspace  VariableName=cd_arm_y  SaveFormat=Timeseries  SampleTime=-1
  ^4 : MATLABFcn  MATLABFcn=u^6
  norm : MATLAB Function  TreatAsAtomicUnit=on
  norm1 : MATLAB Function  TreatAsAtomicUnit=on
  pendiente : Constant  Value=10
  pendiente1 : Constant  Value=2
  pendiente2 : Constant  Value=10
  pendiente3 : Constant
  delta_base : Outport
  wires:
  kskgxm/1 -> Demux/1
  Demux/3 -> Gain/1
  Demux/2 -> Product/2
  Demux/1 -> Product1/2
  Gain/1 -> Mux/3
  Product1/1 -> Mux/1
  Product/1 -> Mux/2
  dist_norm/1 -> Doble funcion Tanh1/1(x), Doble funcion Tanh/1(x)
  pendiente/1 -> Doble funcion Tanh/2(a), Doble funcion Tanh/3(b)
  norm/1(xm_norm) -> Saturation1/1  "xm"
  Sum/1 -> Gain2/1
  Gain1/1 -> Sum/1
  Gain2/1 -> Doble funcion Tanh/5(d), To Workspace1/1, Display1/1, Doble funcion Tanh/4(c)
  Doble funcion Tanh/1(y) -> Product1/1
  pendiente1/1 -> Sum/2
  xm/1 -> FUSE/1  "dist"
  pendiente2/1 -> Doble funcion Tanh1/3(b), Doble funcion Tanh1/2(a)
  Gain3/1 -> To Workspace2/1, Display/1, Doble funcion Tanh1/5(d), Doble funcion Tanh1/4(c)
  Doble funcion Tanh1/1(y) -> Scope/1, Product/1
  Sum1/1 -> Gain3/1
  pendiente3/1 -> Sum1/2
  ^4/1 -> Sum1/1
  norm1/1(xm_norm) -> Saturation/1
  Saturation/1 -> ^4/1
  Saturation1/1 -> Gain1/1
  Mux/1 -> delta_base/1
  FUSE/1 -> norm/1(xm), norm1/1(xm)

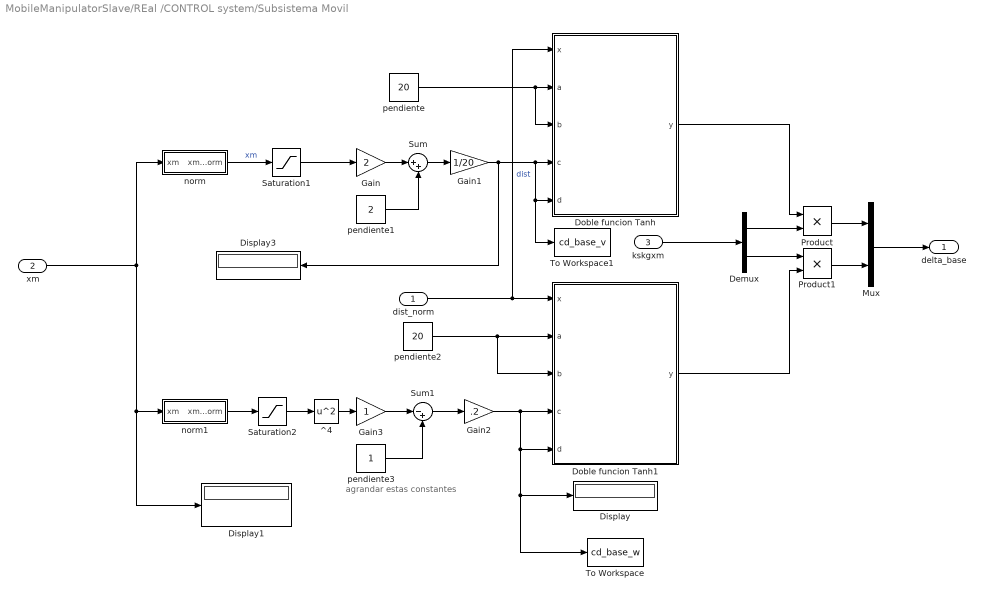
== system MobileManipulatorSlave/REal /CONTROL system/Subsistema Movil ==
  note: agrandar estas constantes
  dist_norm : Inport
  xm : Inport  Port=2
  kskgxm : Inport  Port=3
  Demux : Demux  Outputs=2
  Display : Display
  Display1 : Display
  Display3 : Display
  Doble funcion Tanh : MATLAB Function  TreatAsAtomicUnit=on
  Doble funcion Tanh1 : MATLAB Function  TreatAsAtomicUnit=on
  Gain : Gain  Gain=2
  Gain1 : Gain  Gain=1/20
  Gain2 : Gain  Gain=.2
  Gain3 : Gain
  Mux : Mux  Inputs=2
  Product : Product
  Product1 : Product
  Saturation1 : Saturate  UpperLimit=1  LowerLimit=-1
  Saturation2 : Saturate  UpperLimit=1  LowerLimit=-1
  Sum : Sum  Inputs=|++
  Sum1 : Sum  Inputs=|-+
  To Workspace : ToWorkspace  VariableName=cd_base_w  SaveFormat=Timeseries  SampleTime=-1
  To Workspace1 : ToWorkspace  VariableName=cd_base_v  SaveFormat=Timeseries  SampleTime=-1
  ^4 : MATLABFcn  MATLABFcn=u^2
  norm : MATLAB Function  TreatAsAtomicUnit=on
  norm1 : MATLAB Function  TreatAsAtomicUnit=on
  pendiente : Constant  Value=20
  pendiente1 : Constant  Value=2
  pendiente2 : Constant  Value=20
  pendiente3 : Constant
  delta_base : Outport
  wires:
  kskgxm/1 -> Demux/1
  Demux/1 -> Product/2
  Product/1 -> Mux/1
  Demux/2 -> Product1/1
  Product1/1 -> Mux/2
  Doble funcion Tanh/1(y) -> Product/1
  dist_norm/1 -> Doble funcion Tanh1/1(x), Doble funcion Tanh/1(x)  "dist"
  pendiente/1 -> Doble funcion Tanh/2(a), Doble funcion Tanh/3(b)
  norm/1(xm_norm) -> Saturation1/1  "xm"
  Sum/1 -> Gain1/1
  Gain/1 -> Sum/1
  pendiente1/1 -> Sum/2
  Gain1/1 -> Display3/1, To Workspace1/1, Doble funcion Tanh/5(d), Doble funcion Tanh/4(c)
  pendiente2/1 -> Doble funcion Tanh1/2(a), Doble funcion Tanh1/3(b)
  Gain2/1 -> To Workspace/1, Display/1, Doble funcion Tanh1/5(d), Doble funcion Tanh1/4(c)
  Doble funcion Tanh1/1(y) -> Product1/2
  ^4/1 -> Gain3/1
  Sum1/1 -> Gain2/1
  pendiente3/1 -> Sum1/2
  Gain3/1 -> Sum1/1
  norm1/1(xm_norm) -> Saturation2/1
  Saturation1/1 -> Gain/1
  Saturation2/1 -> ^4/1
  xm/1 -> Display1/1, norm1/1(xm), norm/1(xm)
  Mux/1 -> delta_base/1

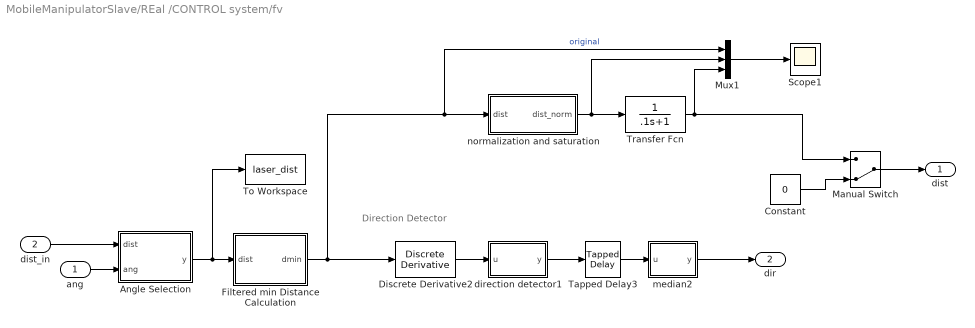
== system MobileManipulatorSlave/REal /CONTROL system/fv ==
  note: Direction Detector
  ang : Inport
  dist_in : Inport  Port=2
  Angle Selection : MATLAB Function  TreatAsAtomicUnit=on
  Constant : Constant  Value=0
  Discrete Derivative2 : simulink/Discrete/Discrete Derivative  gainval=1.0  ICPrevScaledInput=0.0  OutMin=[]  OutMax=[]  OutDataType=fixdt(1, 16)  OutScaling=2^-10  DoSatur=off
  Filtered min Distance Calculation : MATLAB Function  TreatAsAtomicUnit=on
  Manual Switch : ManualSwitch  CurrentSetting=0
  Mux1 : Mux  Inputs=3
  Scope1 : Scope
  Tapped Delay3 : simulink/Discrete/Tapped Delay  vinit=0.0  samptime=-1  NumDelays=6  DelayOrder=Oldest  includeCurrent=off
  To Workspace : ToWorkspace  VariableName=laser_dist  SampleTime=-1
  Transfer Fcn : TransferFcn  Denominator=[.1 1]
  direction detector1 : MATLAB Function  TreatAsAtomicUnit=on
  median2 : MATLAB Function  TreatAsAtomicUnit=on
  normalization and saturation : MATLAB Function  TreatAsAtomicUnit=on
  dist : Outport
  dir : Outport  Port=2
  wires:
  dist_in/1 -> Angle Selection/1(dist)
  Filtered min Distance Calculation/1(dmin) -> normalization and saturation/1(dist), Mux1/1, Discrete Derivative2/1  "original"
  Discrete Derivative2/1 -> direction detector1/1(u)
  direction detector1/1(y) -> Tapped Delay3/1
  median2/1(y) -> dir/1
  Tapped Delay3/1 -> median2/1(u)
  ang/1 -> Angle Selection/2(ang)
  Angle Selection/1(y) -> To Workspace/1, Filtered min Distance Calculation/1(dist)
  normalization and saturation/1(dist_norm) -> Transfer Fcn/1, Mux1/2
  Mux1/1 -> Scope1/1
  Transfer Fcn/1 -> Mux1/3, Manual Switch/1
  Constant/1 -> Manual Switch/2
  Manual Switch/1 -> dist/1

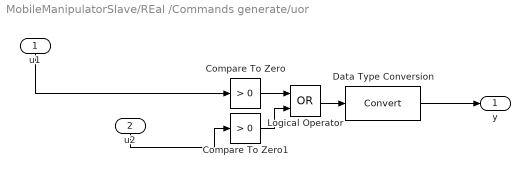
== system MobileManipulatorSlave/REal /Commands generate/uor ==
  u1 : Inport
  u2 : Inport  Port=2
  Compare To Zero : simulink/Logic and Bit Operations/Compare To Zero  relop=>  OutDataTypeStr=boolean
  Compare To Zero1 : simulink/Logic and Bit Operations/Compare To Zero  relop=>  OutDataTypeStr=boolean
  Data Type Conversion : DataTypeConversion
  Logical Operator : Logic  Operator=OR  AllPortsSameDT=off  OutDataTypeStr=boolean
  y : Outport
  wires:
  u2/1 -> Compare To Zero1/1
  Compare To Zero1/1 -> Logical Operator/2
  u1/1 -> Compare To Zero/1
  Compare To Zero/1 -> Logical Operator/1
  Logical Operator/1 -> Data Type Conversion/1
  Data Type Conversion/1 -> y/1

== system MobileManipulatorSlave/REal /CONTROL system/Cinematica Directa2/T2xyz1 ==
  T : Inport
  Demux : Demux  Outputs=3
  MATLAB Fcn : MATLABFcn  MATLABFcn=transl(u)  OutputDimensions=3
  x : Outport
  y : Outport  Port=2
  z : Outport  Port=3
  wires:
  T/1 -> MATLAB Fcn/1
  MATLAB Fcn/1 -> Demux/1
  Demux/1 -> x/1
  Demux/2 -> y/1
  Demux/3 -> z/1

== system MobileManipulatorSlave/REal /CONTROL system/Cinematica Inversa1/Jacobian1 ==
  q : Inport
  MATLAB Function3 : MATLAB Function  TreatAsAtomicUnit=on
  Reshape : Reshape  OutputDimensionality=Row vector (2-D)
  jacob0 : MATLAB Function  TreatAsAtomicUnit=on
  J : Outport
  wires:
  MATLAB Function3/1(J) -> J/1
  q/1 -> Reshape/1
  Reshape/1 -> jacob0/1(in1)
  jacob0/1(out1) -> MATLAB Function3/1(Jc)

== system MobileManipulatorSlave/REal /CONTROL system/Cinematica Inversa1/Metodo Cinematico Inverso ==
  J : Inport
  Inversa sin singularidad : Subsystem
  kin-1 : Outport
  wires:
  J/1 -> Inversa sin singularidad/1(J)
  Inversa sin singularidad/1(invJ) -> kin-1/1

== system MobileManipulatorSlave/REal /CONTROL system/Cinematica Inversa1/Metodo Cinematico Inverso/Inversa sin singularidad ==
  note: Descompone la matriz en SVD y calcula la intersa de S luego recompone la matriz.
      | Si algun termino de la diagonal de S se acerca a 0 lo que hace es no calcular la inversa de ese valor.
      | En su lugar coloca la inversa en 0 (anula el grado de libertad singular)
  J : Inport
  Inversa Segura : MATLAB Function  TreatAsAtomicUnit=on
  Product : Product  Inputs=3  Multiplication=Matrix(*)
  Singular Value Decomposition1 : dspfactors/Singular Value Decomposition  wantv=on  wanterr=off
  transpose : MATLABFcn  MATLABFcn='  Output1D=off
  invJ : Outport
  wires:
  J/1 -> Singular Value Decomposition1/1
  Singular Value Decomposition1/2 -> Inversa Segura/1(u)
  Inversa Segura/1(y) -> Product/2
  Singular Value Decomposition1/1 -> transpose/1
  Product/1 -> invJ/1
  Singular Value Decomposition1/3 -> Product/1
  transpose/1 -> Product/3

== matlab function MobileManipulatorSlave/REal /MATLAB Function ==
  data: sta input; y output; stp input
function y = fcn(sta,stp)
on=[1 1 1];
off=[0 0 0];

if(stp>0)
    y=off;
else
    y=on;
end

== matlab function MobileManipulatorSlave/REal /CONTROL system/MATLAB Function ==
  data: u input; y output; ctr input
function y = fcn(u,ctr)
ctr=1;
v=[.39 0 .113]';
if(ctr>0)
    y = u;
else
    y=v;
end

== matlab function MobileManipulatorSlave/REal /Commands generate/MATLAB Function ==
  data: u input; y output
function y = fcn(u)
if u 
    y=-150;
else
    y=100;
end

== matlab function MobileManipulatorSlave/REal /CONTROL system/Cinematica Directa2/fkine in [cm] ==
  data: in1 input; out1 output
function out1 = fkine(in1)
%#codegen

%    This function was generated by the Symbolic Math Toolbox version 6.1.
%    17-Aug-2017 11:24:58

q1 = in1(1,:);
q2 = in1(2,:);
q3 = in1(3,:);
q4 = in1(4,:);
q5 = in1(5,:);
q6 = in1(6,:);
q7 = in1(7,:);
t2 = cos(q1);
t3 = pi.*(1.0./2.0);
t4 = q6+t3;
t5 = cos(q4);
t6 = sin(q1);
t7 = sin(q3);
t8 = t6.*t7;
t9 = cos(q2);
t10 = cos(q3);
t15 = t2.*t9.*t10;
t11 = t8-t15;
t12 = sin(q2);
t13 = sin(q4);
t14 = sin(q5);
t16 = t5.*t11;
t17 = t2.*t12.*t13;
t18 = t16+t17;
t19 = cos(q5);
t20 = t6.*t10;
t21 = t2.*t7.*t9;
t22 = t20+t21;
t23 = sin(q7);
t24 = sin(t4);
t25 = t11.*t13;
t35 = t2.*t5.*t12;
t26 = t25-t35;
t27 = cos(t4);
t28 = t18.*t19;
t29 = t14.*t22;
t30 = t28+t29;
t36 = t24.*t26;
t37 = t27.*t30;
t31 = t36-t37;
t32 = cos(q7);
t33 = t14.*t18;
t38 = t19.*t22;
t34 = t33-t38;
t39 = t2.*t7;
t40 = t6.*t9.*t10;
t41 = t39+t40;
t42 = t5.*t41;
t46 = t6.*t12.*t13;
t43 = t42-t46;
t44 = t2.*t10;
t48 = t6.*t7.*t9;
t45 = t44-t48;
t47 = t14.*t43;
t59 = t19.*t45;
t49 = t47-t59;
t50 = t13.*t41;
t51 = t5.*t6.*t12;
t52 = t50+t51;
t53 = t24.*t52;
t54 = t19.*t43;
t55 = t14.*t45;
t56 = t54+t55;
t58 = t27.*t56;
t57 = t53-t58;
t60 = t9.*t13;
t61 = t5.*t10.*t12;
t62 = t60+t61;
t63 = t14.*t62;
t64 = t7.*t12.*t19;
t65 = t63+t64;
t66 = t19.*t62;
t73 = t7.*t12.*t14;
t67 = t66-t73;
t68 = t27.*t67;
t69 = t5.*t9;
t74 = t10.*t12.*t13;
t70 = t69-t74;
t71 = t24.*t70;
t72 = t68+t71;
out1 = reshape([-t23.*t34+t31.*t32,t23.*t49-t32.*t57,t23.*t65+t32.*t72,0.0,-t23.*t31-t32.*t34,t23.*t57+t32.*t49,-t23.*t72+t32.*t65,0.0,-t26.*t27-t24.*t30,t27.*t52+t24.*t56,cos(q6).*(-t73+t9.*t13.*t19+t5.*t10.*t12.*t19)+t70.*sin(q6),0.0,t2.*t12.*-1.5e1+t11.*t13.*1.7e1+t24.*t26.*8.0-t23.*t34.*8.0-t27.*t30.*8.0+t31.*t32.*8.0-t2.*t5.*t12.*1.7e1,t6.*t12.*-1.5e1-t13.*t41.*1.7e1+t23.*t49.*8.0-t24.*t52.*8.0+t27.*t56.*8.0-t32.*t57.*8.0-t5.*t6.*t12.*1.7e1,t9.*1.5e1+t5.*t9.*1.7e1+t23.*t65.*8.0+t24.*t70.*8.0+t27.*t67.*8.0+t32.*t72.*8.0-t10.*t12.*t13.*1.7e1+1.2e1,1.0],[4, 4]);

== matlab function MobileManipulatorSlave/REal /CONTROL system/Subsistema Manipulador/Doble funcion Tanh ==
  data: x input; y output; a input; b input; c input; d input
function y   = gap(x,a,b,c,d)%chichon!
%a: pendiente positiva (parte negativa)
%b: pendiente negativa (parte positiva)
%Punto de corte pendiente Positiva= c/a
%Punto de corte pendiente Negativa= b/d
% Redefino los puntos para que corte en c y b 
c=c*a;
d=d*b;
c1=1/2*tanh(a*x+c);
c2=-1/2*tanh(b*x-d);
y = 1-(c1+c2);

== matlab function MobileManipulatorSlave/REal /CONTROL system/fv/direction detector1 ==
  data: u input; y output
function y = fcn(u)
if(u>0)
    y=-1;
elseif(u<0)
    y=1;
else
    y=0;
end

== matlab function MobileManipulatorSlave/REal /CONTROL system/fv/Angle Selection ==
  data: dist input; y output; ang input
function y = fcn(dist,ang)
max=50;%90
n=length(dist);
y=dist;
for i=1:n
    if( (abs(ang(i))>max) || (y(i)==0) )
        y(i)=2;
    end
end

== matlab function MobileManipulatorSlave/REal /CONTROL system/Subsistema Movil/Doble funcion Tanh ==
  data: x input; y output; a input; b input; c input; d input
function y   = bump(x,a,b,c,d)%chichon!
%a: pendiente positiva (parte negativa)
%b: pendiente negativa (parte positiva)
%Punto de corte pendiente Positiva= c/a
%Punto de corte pendiente Negativa= b/d
% Redefino los puntos para que corte en c y b 
c=c*a;
d=d*b;
c1=1/2*tanh(a*x+c);
c2=-1/2*tanh(b*x-d);
y = c1+c2;

== matlab function MobileManipulatorSlave/REal /CONTROL system/Subsistema Movil/Doble funcion Tanh1 ==
  data: x input; y output; a input; b input; c input; d input
function y   = bump(x,a,b,c,d)%chichon!
%a: pendiente positiva (parte negativa)
%b: pendiente negativa (parte positiva)
%Punto de corte pendiente Positiva= c/a
%Punto de corte pendiente Negativa= b/d
% Redefino los puntos para que corte en c y b 
c=c*a;
d=d*b;
c1=1/2*tanh(a*x+c);
c2=-1/2*tanh(b*x-d);
y = c1+c2;

== matlab function MobileManipulatorSlave/REal /CONTROL system/Subsistema Movil/norm1 ==
  data: xm input; xm_norm output
function xm_norm = fcn(xm)
xm_max=0.054;
xm_norm=xm(2)/xm_max;

== matlab function MobileManipulatorSlave/REal /CONTROL system/fv/Filtered min Distance Calculation ==
  data: dmin output; dist input
%Funcion que busca el objeto mas cercano.
%Para estimar la distancia al objeto se toma una vecindad del punto minimo
%si no existen puntos consistentes con el minimo encontrado se elimina 
%y se busco el proximo minimo. 

function dmin  = fcn(dist)
win=10;%ventana en la que se buscan rayos sucesivos.
min_on_win=10;
delta=.02;
tries=50;
max=1.5;
dmin=max;
%busco un minimo consistente en todo el arreglo del laser
% el minimo es consistente si por lo menos 3 rayos sucesivos son similares
%si lo encuentro promedio los rayos similares.
%si no lo encuentro borro el minimo y vuelvo a buscar
%si recorri todo el arreglo y no encontre nada utilizo el maximo
n=length(dist);
while(tries<n)
    [min_dist,i]=min(dist);
    if i<win+1
        i=win+1;
    end
    accum=min_dist;
    k=1;
    for j=1:win
        if (i-j)>0 && (abs(dist(i-j)-min_dist)<delta)
            accum=accum+dist(i-j);
            k=k+1;
        end
        if(i+j)<n && (abs(dist(i+j)-min_dist)<delta)
            accum=accum+dist(i-j);
            k=k+1;
        end
    end
    if(k>min_on_win)
        dmin=accum/k;
        break
    else
        dist(i)=max;%elimino el falso minimo
    end
    tries=tries+1;
end
end

== matlab function MobileManipulatorSlave/REal /CONTROL system/Subsistema Movil/norm ==
  data: xm input; xm_norm output
function xm_norm = fcn(xm)
xm_max=0.05;
xm_norm=xm(1)/xm_max;

== matlab function MobileManipulatorSlave/REal /CONTROL system/fv/median2 ==
  data: u input; y output
function y = fcn(u)
y=median(u);

== matlab function MobileManipulatorSlave/REal /CONTROL system/fv/normalization and saturation ==
  data: dist input; dist_norm output
function dist_norm = factor(dist)
%normaliza la distancia entre 1 y 0
max_dist=1.5; %distancia maxima tenida en cuenta
min_dist=.12; %distancia maxima de acercamiento
dist_norm=1;
if(dist<max_dist)
    dist_norm=dist/max_dist;%normalizacion
end
if(dist<min_dist)
    dist_norm=0;
end

== matlab function MobileManipulatorSlave/REal /CONTROL system/Subsistema Manipulador/norm ==
  data: xm input; xm_norm output
function xm_norm = fcn(xm)
xm_max=0.05;
xm_norm=xm(1)/xm_max;

== matlab function MobileManipulatorSlave/REal /CONTROL system/Subsistema Manipulador/Doble funcion Tanh1 ==
  data: x input; y output; a input; b input; c input; d input
function y   = gap(x,a,b,c,d)%chichon!
%a: pendiente positiva (parte negativa)
%b: pendiente negativa (parte positiva)
%Punto de corte pendiente Positiva= c/a
%Punto de corte pendiente Negativa= b/d
% Redefino los puntos para que corte en c y b 
c=c*a;
d=d*b;
c1=1/2*tanh(a*x+c);
c2=-1/2*tanh(b*x-d);
y = 1-(c1+c2);

== matlab function MobileManipulatorSlave/REal /CONTROL system/Subsistema Manipulador/norm1 ==
  data: xm input; xm_norm output
function xm_norm = fcn(xm)
xm_max=0.054;
xm_norm=xm(2)/xm_max;

== matlab function MobileManipulatorSlave/REal /CONTROL system/Cinematica Inversa1/Jacobian1/MATLAB Function3 ==
  data: Jc input; J output
function J = Jaco(Jc)
J = Jc(1:3,:);
